simulink model "sim"  (R2018a)
settings: Solver=VariableStepAuto  StartTime=0.0  StopTime=10.0  RelTol=1e-3
libraries: fuzblock x1, simulink x1
settings Model: Creator=daniel  LastModifiedBy=daniel

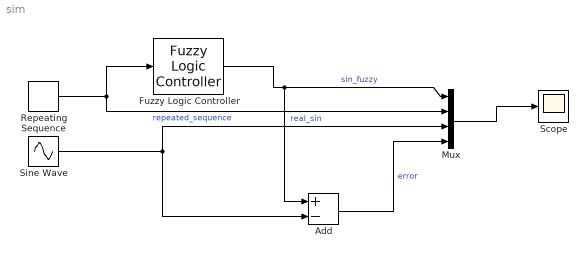
== system sim ==
  Add : Sum  Inputs=+-
  Fuzzy Logic Controller : fuzblock/Fuzzy Logic  Controller  FIS='tipper.fis'  OutputSampleNumber=101  DataType=double  FuzzifiedInputs=off  RuleFiringStrengths=off  RuleOutputs=off  AggregatedOutputs=off  SimulateUsing=Interpreted execution  OutOfRangeInputValueMessage=warning  NoRuleFiredMessage=warning  EmptyOutputFuzzySetMessage=warning
  Mux : Mux
  Repeating Sequence : simulink/Sources/Repeating Sequence  rep_seq_t=IN  rep_seq_y=OUT
  Scope : Scope
  Sine Wave : Sin  Amplitude=0.5  Frequency=2*pi/8  SampleTime=0
  wires:
  Repeating Sequence/1 -> Fuzzy Logic Controller/1, Mux/2  "repeated_sequence"
  Fuzzy Logic Controller/1 -> Add/1, Mux/1  "sin_fuzzy"
  Sine Wave/1 -> Add/2, Mux/3  "real_sin"
  Add/1 -> Mux/4  "error"
  Mux/1 -> Scope/1
